simulink model "musclespindle"  (R2023b)
settings: Solver=FixedStepAuto  StartTime=0.0  StopTime=1  FixedStep=0.0001  RelTol=1e-3
undefined symbols (not defined in the file): b, Kp, Ks, step_time, x_value
settings Model: Creator=muaddib  LastModifiedBy=muaddib

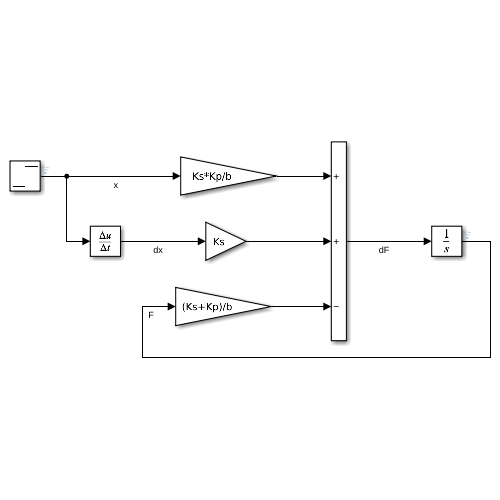
[thumbnail: Simulink's stored preview of the top-level diagram]
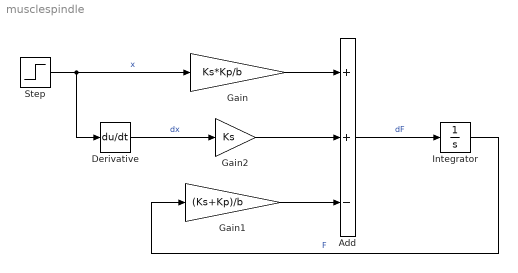
== system musclespindle ==
  Add : Sum  Inputs=++-
  Derivative : Derivative
  Gain : Gain  Gain=Ks*Kp/b
  Gain1 : Gain  Gain=(Ks+Kp)/b
  Gain2 : Gain  Gain=Ks
  Integrator : Integrator
  Step : Step  Time=step_time  After=x_value  SampleTime=0
  wires:
  Step/1 -> Gain/1, Derivative/1  "x"
  Integrator/1 -> Gain1/1  "F"
  Derivative/1 -> Gain2/1  "dx"
  Gain/1 -> Add/1
  Add/1 -> Integrator/1  "dF"
  Gain2/1 -> Add/2
  Gain1/1 -> Add/3
